simulink model "AOO_V1"  (R2019a)
settings: Solver=FixedStepAuto  StartTime=0.0  StopTime=inf  RelTol=1e-3  EnableMultiTasking=on
undefined symbols (not defined in the file or in its folder): D10, D11, D12, D2, D4, D5, D7, D8, D9, PTA0, PTA2, PTB23, PTB9, PTC3, PTC4, PTD0, PTD2, PTD3
libraries: frdmk64flib x9
settings Model: ExtModeTrigDuration=5  Creator=adrso  LastModifiedBy=adrso
settings OptimizationCC: EnhancedBackFolding=on  PassReuseOutputArgsAs=Individual arguments  MaxStackSize=64  OptimizeBlockOrder=speed  DifferentSizesBufferReuse=on  OptimizationCustomize=off
settings DebuggingCC: ParameterTunabilityLossMsg=error
settings HardwareCC: ProdBitPerPointer=32  ProdBitPerSizeT=32  ProdBitPerPtrDiffT=32  ProdLargestAtomicInteger=Long  ProdLargestAtomicFloat=Double  ProdWordSize=32  ProdHWDeviceType=ARM Compatible->ARM Cortex
settings SFSimCC: MATLABDynamicMemAlloc=off
settings RTWCC: SystemTargetFile=ert.tlc  HardwareBoard=NXP FRDM-K64F  TLCOptions="-aInlineSetEventsForThisBaseRateFcn=TLC_FALSE -aSuppressMultiTaskScheduler=TLC_FALSE  -aRateBasedStepFcn=0"  TemplateMakefile=ert_default_tmf  GenerateReport=on  Toolchain=GNU Tools for ARM Embedded Processors  IncludeHyperlinkInReport=on  LaunchReport=on  GenerateTraceInfo=on  GenerateTraceReport=on  GenerateTraceReportSl=on  GenerateTraceReportSf=on  GenerateTraceReportEml=on
settings CodeAppCC: ForceParamTrailComments=on  IgnoreCustomStorageClasses=off  OperatorAnnotations=on  SimulinkDataObjDesc=on  SFDataObjDesc=on  InsertBlockDesc=on

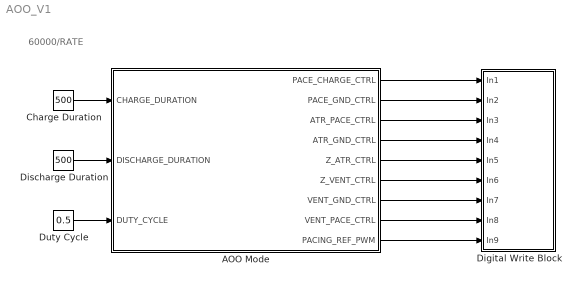
== system AOO_V1 ==
  note: 60000/RATE
  AOO Mode : Stateflow chart  BlockKeywords=__PRM__SERIALIZED__DATA__:Stateflow Chart,Stateflow Diagram  TreatAsAtomicUnit=on
  Charge Duration : Constant  Value=500
  Digital Write Block : Subsystem
  Discharge Duration : Constant  Value=500
  Duty Cycle : Constant  Value=0.5
  wires:
  Charge Duration/1 -> AOO Mode/1(CHARGE_DURATION)
  Discharge Duration/1 -> AOO Mode/2(DISCHARGE_DURATION)
  AOO Mode/9(PACING_REF_PWM) -> Digital Write Block/9(In9)
  AOO Mode/8(VENT_PACE_CTRL) -> Digital Write Block/8(In8)
  AOO Mode/7(VENT_GND_CTRL) -> Digital Write Block/7(In7)
  AOO Mode/6(Z_VENT_CTRL) -> Digital Write Block/6(In6)
  AOO Mode/5(Z_ATR_CTRL) -> Digital Write Block/5(In5)
  AOO Mode/4(ATR_GND_CTRL) -> Digital Write Block/4(In4)
  AOO Mode/3(ATR_PACE_CTRL) -> Digital Write Block/3(In3)
  AOO Mode/2(PACE_GND_CTRL) -> Digital Write Block/2(In2)
  AOO Mode/1(PACE_CHARGE_CTRL) -> Digital Write Block/1(In1)
  Duty Cycle/1 -> AOO Mode/3(DUTY_CYCLE)

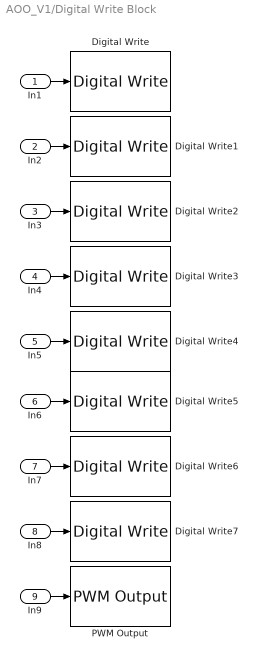
== system AOO_V1/Digital Write Block ==
  In1 : Inport
  In2 : Inport  Port=2
  In3 : Inport  Port=3
  In4 : Inport  Port=4
  In5 : Inport  Port=5
  In6 : Inport  Port=6
  In7 : Inport  Port=7
  In8 : Inport  Port=8
  In9 : Inport  Port=9
  Digital Write : frdmk64flib/Digital Write  Whichpin=PTB9 (D2)
      settings: SourceProductName=Simulink Coder Support Package for NXP FRDM-K64F Board
  Digital Write1 : frdmk64flib/Digital Write  Whichpin=PTD0 (D10)
      settings: SourceProductName=Simulink Coder Support Package for NXP FRDM-K64F Board
  Digital Write2 : frdmk64flib/Digital Write  Whichpin=PTA0 (D8)
      settings: SourceProductName=Simulink Coder Support Package for NXP FRDM-K64F Board
  Digital Write3 : frdmk64flib/Digital Write  Whichpin=PTD2 (D11)
      settings: SourceProductName=Simulink Coder Support Package for NXP FRDM-K64F Board
  Digital Write4 : frdmk64flib/Digital Write  Whichpin=PTB23 (D4)
      settings: SourceProductName=Simulink Coder Support Package for NXP FRDM-K64F Board
  Digital Write5 : frdmk64flib/Digital Write  Whichpin=PTC3 (D7)
      settings: SourceProductName=Simulink Coder Support Package for NXP FRDM-K64F Board
  Digital Write6 : frdmk64flib/Digital Write  Whichpin=PTD3 (D12)
      settings: SourceProductName=Simulink Coder Support Package for NXP FRDM-K64F Board
  Digital Write7 : frdmk64flib/Digital Write  Whichpin=PTC4 (D9)
      settings: SourceProductName=Simulink Coder Support Package for NXP FRDM-K64F Board
  PWM Output : frdmk64flib/PWM Output  Whichpin=PTA2 (D5)  InitialFrequency=2000  InitialDutyCycle=50
      settings: SourceProductName=Simulink Coder Support Package for NXP FRDM-K64F Board
  wires:
  In5/1 -> Digital Write4/1
  In2/1 -> Digital Write1/1
  In6/1 -> Digital Write5/1
  In3/1 -> Digital Write2/1
  In1/1 -> Digital Write/1
  In8/1 -> Digital Write7/1
  In4/1 -> Digital Write3/1
  In7/1 -> Digital Write6/1
  In9/1 -> PWM Output/1

== stateflow chart AOO_V1/AOO Mode ==
  state DISCHARGING
    during:
    %Discharge C22 into ATR
    %Charge C21
    PACE_CHARGE_CTRL = LOW
    PACE_GND_CTRL = HIGH
    ATR_PACE_CTRL = HIGH
    ATR_GND_CTRL = LOW
    Z_ATR_CTRL = LOW
    Z_VENT_CTRL = LOW
    VENT_GND_CTRL = LOW
    VENT_PACE_CTRL = LOW
  state CHARGING
    during:
    %Charge C22
    ATR_PACE_CTRL = LOW
    VENT_PACE_CTRL = LOW
    PACING_REF_PWM = DUTY_CYCLE
    PACE_CHARGE_CTRL = HIGH
    %Discharge C21
    PACE_GND_CTRL = HIGH
    VENT_PACE_CTRL = LOW
    Z_ATR_CTRL = LOW
    Z_VENT_CTRL = LOW
    ATR_PACE_CTRL = LOW
    ATR_GND_CTRL = HIGH
    VENT_GND_CTRL = LOW
  CHARGING -> DISCHARGING : [after(CHARGE_DURATION,msec)]
  (default) -> CHARGING
  DISCHARGING -> CHARGING : [after(DISCHARGE_DURATION,msec)]
  data: CHARGE_DURATION input uint8; DISCHARGE_DURATION input uint8; PACE_CHARGE_CTRL output boolean; PACE_GND_CTRL output boolean; ATR_PACE_CTRL output boolean; ATR_GND_CTRL output boolean; Z_ATR_CTRL output boolean; Z_VENT_CTRL output boolean; VENT_GND_CTRL output boolean; VENT_PACE_CTRL output boolean; PACING_REF_PWM output boolean; LOW local boolean =0; HIGH local boolean =1; DUTY_CYCLE input uint8
